simulink model "model"  (R2025b)
settings: Solver=FixedStepAuto  StartTime=0.0  StopTime=25  FixedStep=0.01  RelTol=1e-3
undefined symbols (not defined in the file or in its folder): n1, n2
settings Model: Creator=Atread  LastModifiedBy=Atread
settings OptimizationCC: OptimizeBlockIOStorage=off  OptimizeDataStoreBuffers=off  BusAssignmentInplaceUpdate=off
settings DebuggingCC: SFUnexpectedBacktrackingDiag=warning  SFNoUnconditionalDefaultTransitionDiag=warning
settings RTWCC: GenerateReport=on  BuildConfiguration=Debug  LaunchReport=on
settings CodeAppCC: ForceParamTrailComments=on  MATLABSourceComments=on  EnableCustomComments=on
settings GRTTargetCC: MultiInstanceErrorCode=Warning  CombineSignalStateStructs=on  SupportVariableSizeSignals=on

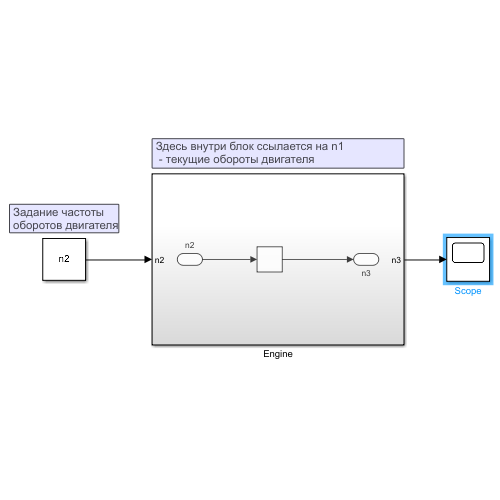
[thumbnail: Simulink's stored preview of the top-level diagram]
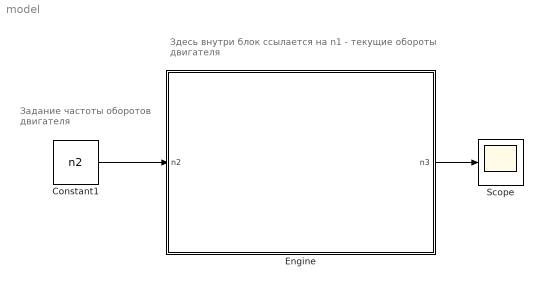
== system model ==
  note: Здесь внутри блок ссылается на n1
      |  - текущие обороты двигателя
  note: Задание частоты
      | оборотов двигателя
  Constant1 : Constant  Value=n2
  Engine : Subsystem
  Scope : Scope
      settings: ActiveDisplayYMinimum=-1053.6965219537606  ActiveDisplayYMaximum=3401.1495767848919
  wires:
  Constant1/1 -> Engine/1(n2)
  Engine/1(n3) -> Scope/1

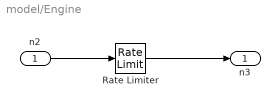
== system model/Engine ==
  n2 : Inport
  Rate Limiter : RateLimiter  RisingSlewLimit=250  FallingSlewLimit=-250  SampleTimeMode=inherited  InitialCondition=n1
  n3 : Outport
  wires:
  n2/1 -> Rate Limiter/1
  Rate Limiter/1 -> n3/1
